simulink model "airspeed_pitch"  (R2017a)
settings: Solver=VariableStepAuto  StartTime=0.0  StopTime=100  RelTol=1e-3
values from neighbouring files (symbols this model uses):
  a_theta1 = -P.rho*Va^2*P.c*P.S_wing/(2*P.Jy)*P.C_m_q*P.c/(2*Va)    [computeRollGains.m]    (also in compute_gains.m)
  a_theta2 = -P.rho*Va^2*P.c*P.S_wing*P.C_m_alpha/(2*P.Jy)    [computeRollGains.m]    (also in compute_gains.m)
  a_theta3 = P.rho*Va^2*P.c*P.S_wing/(2*P.Jy)*P.C_m_delta_e    [computeRollGains.m]    (also in compute_gains.m)
  a_V1 = P.rho*Va*P.S_wing/P.mass*(P.C_D_0 + P.C_D_alpha*alpha +      P.C_D_delta_e*delta_e) + P.rho*P.S_wing*P.C_prop*Va/P.mass    [computeRollGains.m]    (also in compute_gains.m = P.rho*Va*P.S_wing/P.mass*(P.C_D_0 + P.C_D_alpha*alpha_trim +)
  delta_e_max = 45*pi/180    (= 0.785398163397)    [computeRollGains.m]    (also in compute_gains.m = 0.523598775598)
  P = struct    [vehicle_params.m]
settings Model: Creator=pizzaslayer  LastModifiedBy=pizzaslayer

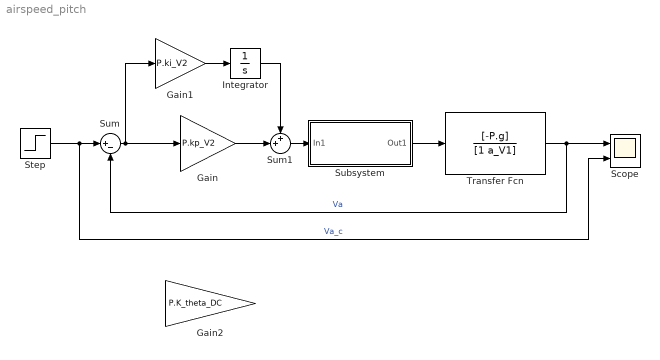
== system airspeed_pitch ==
  Gain : Gain  Gain=P.kp_V2
  Gain1 : Gain  Gain=P.ki_V2
  Gain2 : Gain  Gain=P.K_theta_DC
  Integrator : Integrator
  Scope : Scope  NumInputPorts=2
  Step : Step  Time=0  After=5  SampleTime=0
  Subsystem : Subsystem
  Sum : Sum  Inputs=|+-
  Sum1 : Sum  Inputs=++|
  Transfer Fcn : TransferFcn  Numerator=[-P.g]  Denominator=[1 a_V1]
  wires:
  Step/1 -> Scope/2, Sum/1  "Va_c"
  Gain1/1 -> Integrator/1
  Sum/1 -> Gain/1, Gain1/1
  Integrator/1 -> Sum1/1
  Gain/1 -> Sum1/2
  Transfer Fcn/1 -> Sum/2, Scope/1  "Va"
  Sum1/1 -> Subsystem/1(In1)
  Subsystem/1(Out1) -> Transfer Fcn/1

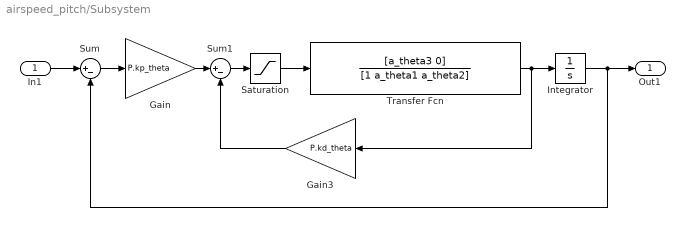
== system airspeed_pitch/Subsystem ==
  In1 : Inport
  Gain : Gain  Gain=P.kp_theta
  Gain3 : Gain  Gain=P.kd_theta
  Integrator : Integrator
  Saturation : Saturate  UpperLimit=delta_e_max  LowerLimit=-delta_e_max
  Sum : Sum  Inputs=|+-
  Sum1 : Sum  Inputs=|+-
  Transfer Fcn : TransferFcn  Numerator=[a_theta3 0]  Denominator=[1 a_theta1 a_theta2]
  Out1 : Outport
  wires:
  In1/1 -> Sum/1
  Transfer Fcn/1 -> Integrator/1, Gain3/1
  Gain3/1 -> Sum1/2
  Sum1/1 -> Saturation/1
  Gain/1 -> Sum1/1
  Sum/1 -> Gain/1
  Integrator/1 -> Out1/1, Sum/2
  Saturation/1 -> Transfer Fcn/1
